simulink model "Quanser_simulink"  (R2022a)
settings: Solver=VariableStepAuto  StartTime=0.0  StopTime=10  RelTol=1e-3
libraries: simulink_extras x3
settings Model: PacingRate=3  Creator=Administrator  LastModifiedBy=mluser
settings DebuggingCC: UnconnectedInputMsg=warning  UnconnectedOutputMsg=warning  UnconnectedLineMsg=warning
settings RTWCC: DLArmComputeVersion=19.05

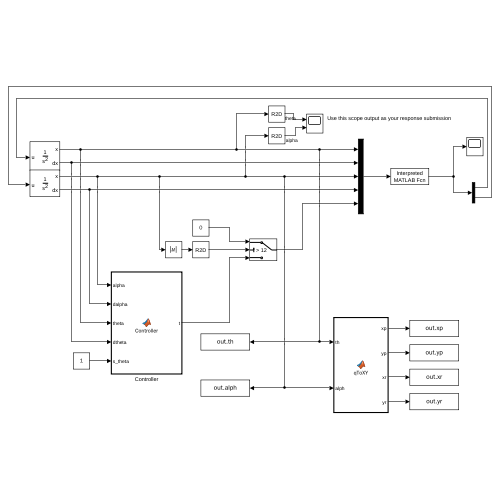
[thumbnail: Simulink's stored preview of the top-level diagram]
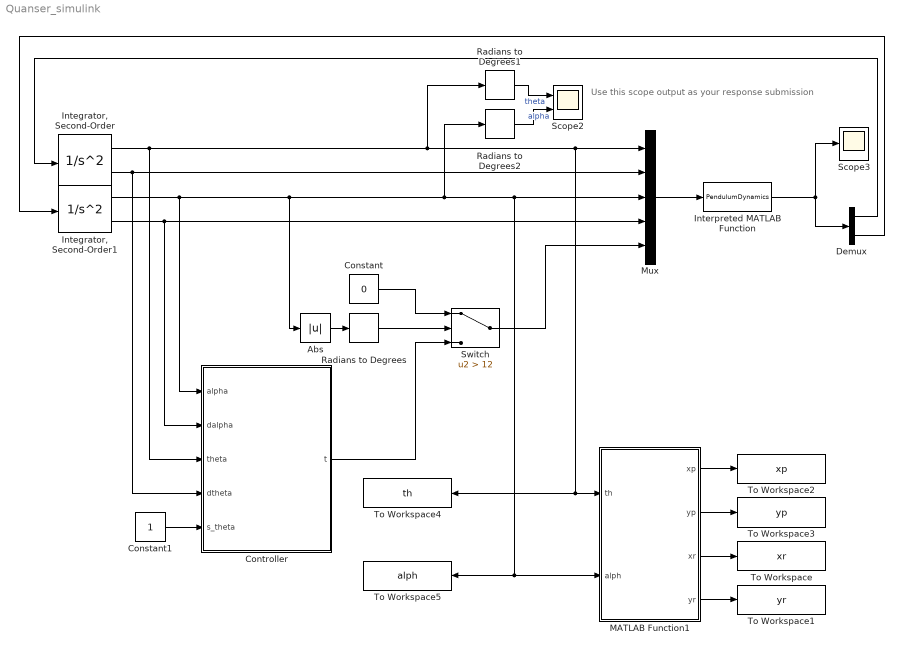
== system Quanser_simulink ==
  note: Use this scope output as your response submission
  Abs : Abs  SaturateOnIntegerOverflow=off
  Constant : Constant  Value=0
  Constant1 : Constant
  Controller : MATLAB Function  TreatAsAtomicUnit=on
  Demux : Demux  Outputs=2
  "Integrator, Second-Order" : SecondOrderIntegrator  ICX=0
  "Integrator, Second-Order1" : SecondOrderIntegrator  ICX=0.1
  Interpreted MATLAB Function : MATLABFcn  MATLABFcn=PendulumDynamics  OutputDimensions=2
  MATLAB Function1 : MATLAB Function  TreatAsAtomicUnit=on
  Mux : Mux  Inputs=5
  Radians to Degrees : simulink_extras/Transformations/Radians to Degrees
  Radians to Degrees1 : simulink_extras/Transformations/Radians to Degrees
  Radians to Degrees2 : simulink_extras/Transformations/Radians to Degrees
  Scope2 : Scope  NumInputPorts=2
  Scope3 : Scope
  Switch : Switch  Criteria=u2 > Threshold  Threshold=12  SaturateOnIntegerOverflow=off  InputSameDT=off
  To Workspace : ToWorkspace  VariableName=xr  SaveFormat=Structure With Time  SampleTime=-1
  To Workspace1 : ToWorkspace  VariableName=yr  SaveFormat=Structure With Time  SampleTime=-1
  To Workspace2 : ToWorkspace  VariableName=xp  SaveFormat=Structure With Time  SampleTime=-1
  To Workspace3 : ToWorkspace  VariableName=yp  SaveFormat=Structure With Time  SampleTime=-1
  To Workspace4 : ToWorkspace  VariableName=th  SaveFormat=Structure With Time  SampleTime=-1
  To Workspace5 : ToWorkspace  VariableName=alph  SaveFormat=Structure With Time  SampleTime=-1
  wires:
  Demux/1 -> "Integrator, Second-Order"/1
  Demux/2 -> "Integrator, Second-Order1"/1
  Interpreted MATLAB Function/1 -> Scope3/1, Demux/1
  Mux/1 -> Interpreted MATLAB Function/1
  "Integrator, Second-Order"/2 -> Mux/2, Controller/4(dtheta)
  "Integrator, Second-Order1"/2 -> Controller/2(dalpha), Mux/4
  Switch/1 -> Mux/5
  MATLAB Function1/3(xr) -> To Workspace/1
  MATLAB Function1/4(yr) -> To Workspace1/1
  MATLAB Function1/2(yp) -> To Workspace3/1
  MATLAB Function1/1(xp) -> To Workspace2/1
  Abs/1 -> Radians to Degrees/1
  Radians to Degrees/1 -> Switch/2
  Constant/1 -> Switch/1
  Constant1/1 -> Controller/5(s_theta)
  Controller/1(t) -> Switch/3
  "Integrator, Second-Order"/1 -> To Workspace4/1, MATLAB Function1/1(th), Mux/1, Radians to Degrees1/1, Controller/3(theta)
  "Integrator, Second-Order1"/1 -> Controller/1(alpha), Abs/1, MATLAB Function1/2(alph), To Workspace5/1, Mux/3, Radians to Degrees2/1
  Radians to Degrees1/1 -> Scope2/1  "theta"
  Radians to Degrees2/1 -> Scope2/2  "alpha"

== matlab function Quanser_simulink/MATLAB Function1 ==
  data: th input; xp output; yp output; alph input; xr output; yr output
function [xp, yp, xr, yr] = qToXY(th,alph)
    R01 = Rotz(th); %from frame 0 to frame 1
    R10 = transpose(R01); %from 1 to Inertial
    R12 = Rotx(alph);
    R02 = R12*R01; %from frame 0 to frame 2 
    R20 = transpose(R02); %from 2 to Inertial
    
    Lr = 0.085;
    Lp = 0.129;
    
    rArm_1 = (Lr/2)*[1; 0; 0];
    rArm_0 = R10*rArm_1;
    xr = rArm_0(1);
    yr = rArm_0(2);
    
    rPen_2 =(Lp/2)*[0;0;1];
    rPen_0 = rArm_0*2+R20*rPen_2;
    xp = rPen_0(1);
    yp = rPen_0(2);
end

%% Helper Functions 
function A = Rotx(th)
    A = [1 0        0;...
         0 cos(th)  sin(th);...
         0 -sin(th)  cos(th)];
end
 
function A = Roty(th)
    A = [cos(th)  0   -sin(th);...
         0        1   0;...
         sin(th)  0   cos(th)];
end 

function A = Rotz(th)
    A = [cos(th)   sin(th) 0;... 
         -sin(th)  cos(th) 0;...
         0        0        1];
end

== matlab function Quanser_simulink/Controller ==
  data: alpha input; t output; dalpha input; theta input; dtheta input; s_theta input
function t = Controller(alpha, dalpha, theta, dtheta, s_theta)
    % CODE HERE
    Input = [theta; alpha; dtheta; dalpha];
    K = [-5.7735 196.0114 -7.2777 24.6382];
    
    Kr=-5.7735;
    t = s_theta*Kr-K*Input;
end
